simulink library "BPN_lib"  (Simulink 7.4)
settings: Solver=ode45  StartTime=0.0  StopTime=10.0  RelTol=1e-3
values from neighbouring files (symbols this model uses):
  BPNc_fac_ChaPowCurLim = mpt.Parameter    [BPN_CAL.m]
  BPNc_fac_DchPowCurLim = mpt.Parameter    [BPN_CAL.m]
  BPNc_i2_ContiChaCurLim_Max = mpt.Parameter    [BPN_CAL.m]
  BPNc_i2_ContiDchCurLim_Max = mpt.Parameter    [BPN_CAL.m]
  BPNc_i_ContiChaCurLim_Max = mpt.Parameter    [BPN_CAL.m]
  BPNc_i_ContiDchCurLim_Max = mpt.Parameter    [BPN_CAL.m]
  BPNc_i_NorChaCurLim_Max = mpt.Parameter    [BPN_CAL.m]
  BPNc_i_NorDchCurLim_Max = mpt.Parameter    [BPN_CAL.m]
  BPNc_i_PackCurMeasAlwd = mpt.Parameter    [BPN_CAL.m]
  BPNc_i_SafeChaCurLim_Max = mpt.Parameter    [BPN_CAL.m]
  BPNc_i_SafeDchCurLim_Max = mpt.Parameter    [BPN_CAL.m]
  BPNc_pct_CurLimFac_warn = mpt.Parameter    [BPN_CAL.m]
  BPNc_pct_PackSocOver_fatal = mpt.Parameter    [BPN_CAL.m]
  BPNc_pct_PackSocOver_fault = mpt.Parameter    [BPN_CAL.m]
  BPNc_pct_PackSocOver_warn = mpt.Parameter    [BPN_CAL.m]
  BPNc_pct_PackSocUnder_fatal = mpt.Parameter    [BPN_CAL.m]
  BPNc_pct_PackSocUnder_fault = mpt.Parameter    [BPN_CAL.m]
  BPNc_pct_PackSocUnder_warn = mpt.Parameter    [BPN_CAL.m]
  BPNc_pct_PowLimfac_fatal = mpt.Parameter    [BPN_CAL.m]
  BPNc_pct_PowLimfac_warn = mpt.Parameter    [BPN_CAL.m]
  BPNc_r_CtrRes_fault = mpt.Parameter    [BPN_CAL.m]
  BPNc_r_PackInResThrld = mpt.Parameter    [BPN_CAL.m]
  BPNc_t_PackTemp_Mean = mpt.Parameter    [BPN_CAL.m]
  BPNc_v_CellVoltDif_fault = mpt.Parameter    [BPN_CAL.m]
  BPNc_v_CellVoltDif_warn = mpt.Parameter    [BPN_CAL.m]
  BPNc_v_CellVoltOver_fatal = mpt.Parameter    [BPN_CAL.m]
  BPNc_v_CellVoltOver_fault = mpt.Parameter    [BPN_CAL.m]
  BPNc_v_CellVoltOver_warn = mpt.Parameter    [BPN_CAL.m]
  BPNc_v_CellVoltUnder_fatal = mpt.Parameter    [BPN_CAL.m]
  BPNc_v_CellVoltUnder_fault = mpt.Parameter    [BPN_CAL.m]
  BPNc_v_CellVoltUnder_warn = mpt.Parameter    [BPN_CAL.m]
  BPNc_v_LowOPerVolt = mpt.Parameter    [BPN_CAL.m]
  BPNc_v_PackVoltDrop_fatal = mpt.Parameter    [BPN_CAL.m]
  BPNc_v_PackVoltOver_fatal = mpt.Parameter    [BPN_CAL.m]
  BPNc_v_PackVoltOver_fault = mpt.Parameter    [BPN_CAL.m]
  BPNc_v_PackVoltOver_warn = mpt.Parameter    [BPN_CAL.m]
  BPNc_v_PackVoltUnder_fatal = mpt.Parameter    [BPN_CAL.m]
  BPNc_v_PackVoltUnder_fault = mpt.Parameter    [BPN_CAL.m]
  BPNc_v_PackVoltUnder_warn = mpt.Parameter    [BPN_CAL.m]
  BPNc_v_VoltDifThrld = mpt.Parameter    [BPN_CAL.m]
  BPNy_DiagAcvnCtlCtrSt = mpt.Parameter    [BPN_CAL.m]
  BPNz_DiagAcvnCtlId = mpt.Parameter    [BPN_CAL.m]
  BSCx_BCU_State = mpt.Parameter    [BPN_CAL.m]
undefined symbols (not defined in the file or in its folder): BMS_Const_TickTm_s, BPNm_mode_DiaCtlAcv, PACK_Const_CellNumOfMdl, PACK_Const_MdlNumOfPack
libraries: Defined_Functionality x12, simulink x4
(part 2 of 2)

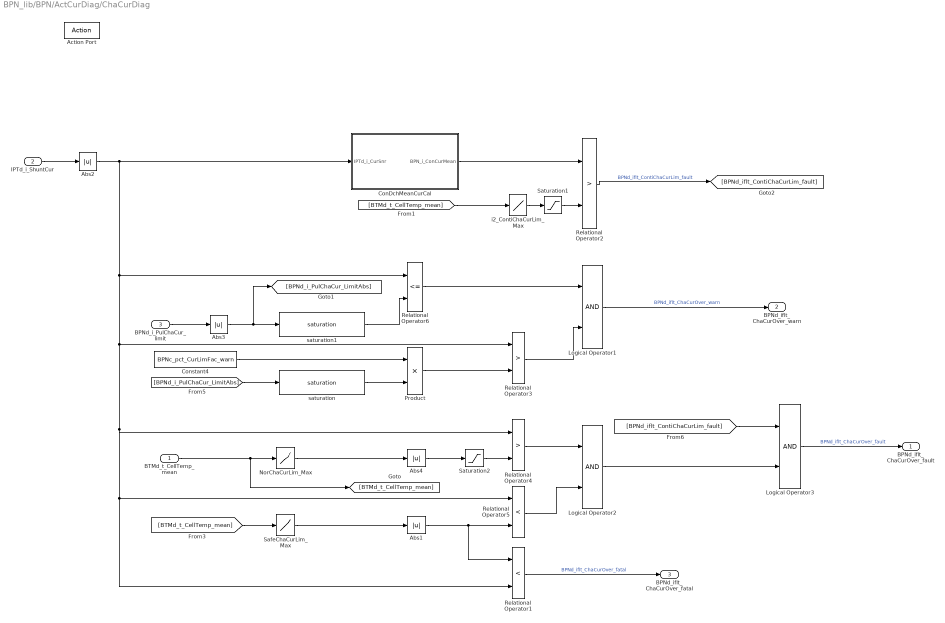
== system BPN_lib/BPN/ActCurDiag/ChaCurDiag ==
  BTMd_t_CellTemp_mean : Inport
  IPTd_i_ShuntCur : Inport  Port=2
  BPNd_i_PulChaCur_limit : Inport  Port=3
  Action Port : ActionPort
  Abs1 : Abs  OutDataType=fixdt(1, 16)  OutScaling=2^0
  Abs2 : Abs
  Abs3 : Abs
  Abs4 : Abs  OutDataType=fixdt(1, 16)  OutScaling=2^0
  ConDchMeanCurCal : Subsystem
  Constant4 : Constant  Value=BPNc_pct_CurLimFac_warn
  Logical Operator1 : Logic  AllPortsSameDT=off  OutDataTypeMode=boolean  OutDataTypeStr=boolean
  Logical Operator2 : Logic  AllPortsSameDT=off  OutDataTypeMode=boolean  OutDataTypeStr=boolean
  Logical Operator3 : Logic  AllPortsSameDT=off  OutDataTypeMode=boolean  OutDataTypeStr=boolean
  NorChaCurLim_Max : Lookup  InputValues=BPNc_t_PackTemp_Mean  Table=BPNc_i_NorChaCurLim_Max  LookUpMeth=Interpolation-Use End Values
  Product : Product  RndMeth=Zero
  Relational Operator1 : RelationalOperator  Operator=<  LogicOutDataTypeMode=boolean  OutDataTypeStr=boolean
  Relational Operator2 : RelationalOperator  Operator=>  LogicOutDataTypeMode=boolean  OutDataTypeStr=boolean
  Relational Operator3 : RelationalOperator  Operator=>  LogicOutDataTypeMode=boolean  OutDataTypeStr=boolean
  Relational Operator4 : RelationalOperator  Operator=>  LogicOutDataTypeMode=boolean  OutDataTypeStr=boolean
  Relational Operator5 : RelationalOperator  Operator=<  LogicOutDataTypeMode=boolean  OutDataTypeStr=boolean
  Relational Operator6 : RelationalOperator  Operator=<=  LogicOutDataTypeMode=boolean  OutDataTypeStr=boolean
  SafeChaCurLim_Max : Lookup  InputValues=BPNc_t_PackTemp_Mean  Table=BPNc_i_SafeChaCurLim_Max  LookUpMeth=Interpolation-Use End Values
  Saturation1 : Saturate  UpperLimit=46000  LowerLimit=100
  Saturation2 : Saturate  UpperLimit=300  LowerLimit=15
  i2_ContiChaCurLim_Max : Lookup  InputValues=BPNc_t_PackTemp_Mean  Table=BPNc_i2_ContiChaCurLim_Max  LookUpMeth=Interpolation-Use End Values
  saturation : Defined_Functionality/saturation  SystemSampleTime=-1  upper_limit=300  lower_limit=15
      settings: AttributesFormatString=[UPPER_LIMIT=%<upper_limit>]\n[LOWER_LIMIT=%<lower_limit>]
  saturation1 : Defined_Functionality/saturation  SystemSampleTime=-1  upper_limit=500  lower_limit=15
      settings: AttributesFormatString=[UPPER_LIMIT=%<upper_limit>]\n[LOWER_LIMIT=%<lower_limit>]
  BPNd_iflt_ChaCurOver_fault : Outport
  BPNd_iflt_ChaCurOver_warn : Outport  Port=2
  BPNd_iflt_ChaCurOver_fatal : Outport  Port=3
  wires:
  Abs2/1 -> Relational Operator6/1, Relational Operator3/1, Relational Operator1/2, Relational Operator5/1, Relational Operator4/1, ConDchMeanCurCal/1(IPTd_i_CurSnr)
  [BPNd_iflt_ContiChaCurLim_fault] -> Logical Operator3/1
  Logical Operator3/1 -> BPNd_iflt_ChaCurOver_fault/1  "BPNd_iflt_ChaCurOver_fault"
  Logical Operator2/1 -> Logical Operator3/2
  Relational Operator2/1 -> [BPNd_iflt_ContiChaCurLim_fault]  "BPNd_iflt_ContiChaCurLim_fault"
  Abs1/1 -> Relational Operator5/2, Relational Operator1/1
  Abs4/1 -> Saturation2/1
  saturation1/1 -> Relational Operator6/2
  Saturation2/1 -> Relational Operator4/2
  Saturation1/1 -> Relational Operator2/2
  saturation/1 -> Product/2
  ConDchMeanCurCal/1(BPN_i_ConCurMean) -> Relational Operator2/1
  Relational Operator5/1 -> Logical Operator2/2
  Relational Operator4/1 -> Logical Operator2/1
  SafeChaCurLim_Max/1 -> Abs1/1
  Logical Operator1/1 -> BPNd_iflt_ChaCurOver_warn/1  "BPNd_iflt_ChaCurOver_warn"
  Relational Operator3/1 -> Logical Operator1/2
  Relational Operator6/1 -> Logical Operator1/1
  [BPNd_i_PulChaCur_LimitAbs] -> saturation/1
  Abs3/1 -> saturation1/1, [BPNd_i_PulChaCur_LimitAbs]
  Product/1 -> Relational Operator3/2
  Constant4/1 -> Product/1
  BPNd_i_PulChaCur_limit/1 -> Abs3/1
  [BTMd_t_CellTemp_mean] -> SafeChaCurLim_Max/1
  [BTMd_t_CellTemp_mean] -> i2_ContiChaCurLim_Max/1
  BTMd_t_CellTemp_mean/1 -> [BTMd_t_CellTemp_mean], NorChaCurLim_Max/1
  NorChaCurLim_Max/1 -> Abs4/1
  IPTd_i_ShuntCur/1 -> Abs2/1
  i2_ContiChaCurLim_Max/1 -> Saturation1/1
  Relational Operator1/1 -> BPNd_iflt_ChaCurOver_fatal/1  "BPNd_iflt_ChaCurOver_fatal"

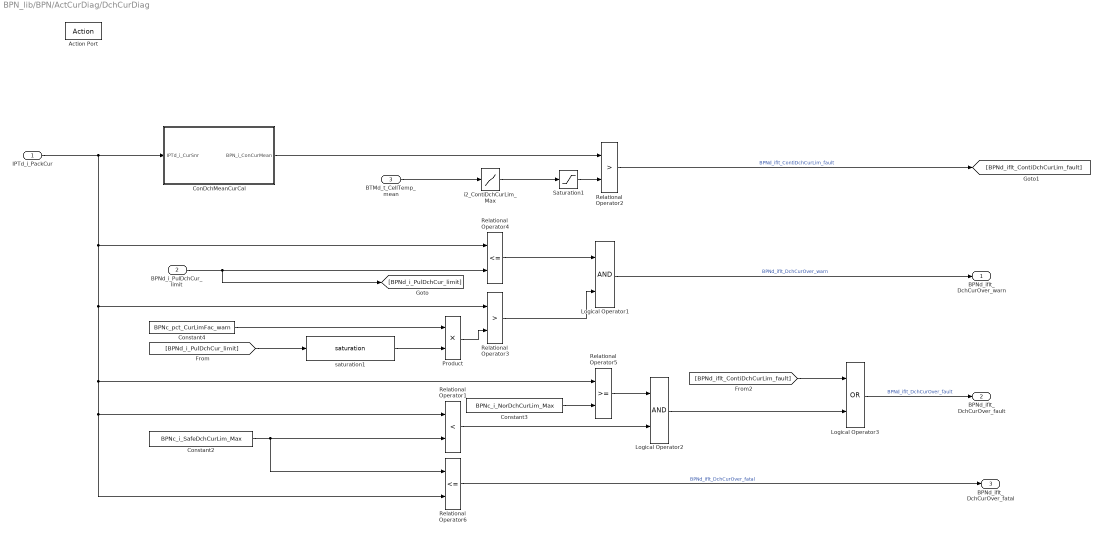
== system BPN_lib/BPN/ActCurDiag/DchCurDiag ==
  IPTd_i_PackCur : Inport  DataType=single  OutDataTypeStr=single
  BPNd_i_PulDchCur_limit : Inport  Port=2
  BTMd_t_CellTemp_mean : Inport  Port=3
  Action Port : ActionPort
  ConDchMeanCurCal : Subsystem
  Constant2 : Constant  Value=BPNc_i_SafeDchCurLim_Max  OutDataTypeMode=single  OutDataTypeStr=single
  Constant3 : Constant  Value=BPNc_i_NorDchCurLim_Max  OutDataTypeMode=single  OutDataTypeStr=single
  Constant4 : Constant  Value=BPNc_pct_CurLimFac_warn
  Logical Operator1 : Logic  AllPortsSameDT=off  OutDataTypeMode=boolean  OutDataTypeStr=boolean
  Logical Operator2 : Logic  AllPortsSameDT=off  OutDataTypeMode=boolean  OutDataTypeStr=boolean
  Logical Operator3 : Logic  Operator=OR  AllPortsSameDT=off  OutDataTypeMode=boolean  OutDataTypeStr=boolean
  Product : Product  RndMeth=Zero
  Relational Operator1 : RelationalOperator  Operator=<  LogicOutDataTypeMode=boolean  OutDataTypeStr=boolean
  Relational Operator2 : RelationalOperator  Operator=>  LogicOutDataTypeMode=boolean  OutDataTypeStr=boolean
  Relational Operator3 : RelationalOperator  Operator=>  LogicOutDataTypeMode=boolean  OutDataTypeStr=boolean
  Relational Operator4 : RelationalOperator  Operator=<=  LogicOutDataTypeMode=boolean  OutDataTypeStr=boolean
  Relational Operator5 : RelationalOperator  LogicOutDataTypeMode=boolean  OutDataTypeStr=boolean
  Relational Operator6 : RelationalOperator  Operator=<=  LogicOutDataTypeMode=boolean  OutDataTypeStr=boolean
  Saturation1 : Saturate  UpperLimit=90000  LowerLimit=5
  i2_ContiDchCurLim_Max : Lookup  InputValues=BPNc_t_PackTemp_Mean  Table=BPNc_i2_ContiDchCurLim_Max  LookUpMeth=Interpolation-Use End Values
  saturation1 : Defined_Functionality/saturation  SystemSampleTime=-1  upper_limit=300  lower_limit=15
      settings: AttributesFormatString=[UPPER_LIMIT=%<upper_limit>]\n[LOWER_LIMIT=%<lower_limit>]
  BPNd_iflt_DchCurOver_warn : Outport
  BPNd_iflt_DchCurOver_fault : Outport  Port=2
  BPNd_iflt_DchCurOver_fatal : Outport  Port=3
  wires:
  saturation1/1 -> Product/2
  [BPNd_i_PulDchCur_limit] -> saturation1/1
  IPTd_i_PackCur/1 -> Relational Operator6/2, Relational Operator1/1, Relational Operator5/1, Relational Operator3/1, Relational Operator4/1, ConDchMeanCurCal/1(IPTd_i_CurSnr)
  [BPNd_iflt_ContiDchCurLim_fault] -> Logical Operator3/1
  Logical Operator3/1 -> BPNd_iflt_DchCurOver_fault/1  "BPNd_iflt_DchCurOver_fault"
  Logical Operator2/1 -> Logical Operator3/2
  Constant3/1 -> Relational Operator5/2
  Relational Operator2/1 -> [BPNd_iflt_ContiDchCurLim_fault]  "BPNd_iflt_ContiDchCurLim_fault"
  ConDchMeanCurCal/1(BPN_i_ConCurMean) -> Relational Operator2/1
  Saturation1/1 -> Relational Operator2/2
  Relational Operator6/1 -> BPNd_iflt_DchCurOver_fatal/1  "BPNd_iflt_DchCurOver_fatal"
  Relational Operator1/1 -> Logical Operator2/2
  Relational Operator5/1 -> Logical Operator2/1
  Constant2/1 -> Relational Operator6/1, Relational Operator1/2
  Logical Operator1/1 -> BPNd_iflt_DchCurOver_warn/1  "BPNd_iflt_DchCurOver_warn"
  Relational Operator3/1 -> Logical Operator1/2
  Relational Operator4/1 -> Logical Operator1/1
  BPNd_i_PulDchCur_limit/1 -> [BPNd_i_PulDchCur_limit], Relational Operator4/2
  Product/1 -> Relational Operator3/2
  Constant4/1 -> Product/1
  i2_ContiDchCurLim_Max/1 -> Saturation1/1
  BTMd_t_CellTemp_mean/1 -> i2_ContiDchCurLim_Max/1

== system BPN_lib/BPN/ActCurDiag/Subsystem ==
  BPNd_i_PulDchCur_limit : Inport
  BPNd_i_PulChaCur_limit : Inport  Port=2
  Abs : Abs  OutDataType=fixdt(1, 16)  OutScaling=2^0
  Bus Creator : BusCreator  Inputs=2
  Bus Creator1 : BusCreator  Inputs=2
  MinMax : MinMax  Function=max
  MinMax1 : MinMax
  Selector : Selector  InputPortWidth=11  IndexOptions=Index vector (dialog)  Indices=2:11  OutputSizes=1
  Selector1 : Selector  InputPortWidth=11  IndexOptions=Index vector (dialog)  Indices=2:11  OutputSizes=1
  Unit Delay : UnitDelay  SampleTime=-1
  Unit Delay1 : UnitDelay  SampleTime=-1
  BPN_i_PulDchCur_limit : Outport
  BPN_i_PulChaCur_LimitAbs : Outport  Port=2
  wires:
  Abs/1 -> BPN_i_PulChaCur_LimitAbs/1
  MinMax1/1 -> Abs/1
  MinMax/1 -> BPN_i_PulDchCur_limit/1
  BPNd_i_PulChaCur_limit/1 -> Bus Creator1/2
  Unit Delay1/1 -> Bus Creator1/1
  Bus Creator1/1 -> Selector1/1
  BPNd_i_PulDchCur_limit/1 -> Bus Creator/2
  Unit Delay/1 -> Bus Creator/1
  Bus Creator/1 -> Selector/1
  Selector1/1 -> MinMax1/1, Unit Delay1/1
  Selector/1 -> MinMax/1, Unit Delay/1

== system BPN_lib/BPN/ActPowDiag/PulChaPower_Diagnosic ==
  BPNd_pow_PackActPower : Inport
  BPNd_pow_PulChaPower_limit : Inport  Port=2
  Action Port : ActionPort
  Abs : Abs
  Abs1 : Abs
  Constant2 : Constant  Value=BPNc_pct_PowLimfac_warn
  Constant3 : Constant  Value=BPNc_pct_PowLimfac_fatal
  Logical Operator1 : Logic  AllPortsSameDT=off  OutDataTypeMode=boolean  OutDataTypeStr=boolean
  Product2 : Product  RndMeth=Zero
  Product3 : Product  RndMeth=Zero
  Relational Operator2 : RelationalOperator  Operator=<  LogicOutDataTypeMode=boolean  OutDataTypeStr=boolean
  Relational Operator3 : RelationalOperator  LogicOutDataTypeMode=boolean  OutDataTypeStr=boolean
  Relational Operator4 : RelationalOperator  Operator=<=  LogicOutDataTypeMode=boolean  OutDataTypeStr=boolean
  Relational Operator6 : RelationalOperator  Operator=>  LogicOutDataTypeMode=boolean  OutDataTypeStr=boolean
  saturation : Defined_Functionality/saturation  SystemSampleTime=-1  upper_limit=500000  lower_limit=10000
      settings: AttributesFormatString=[UPPER_LIMIT=%<upper_limit>]\n[LOWER_LIMIT=%<lower_limit>]
  signal_debug : Defined_Functionality/signal_debug  SystemSampleTime=-1  debug_switch=BPNc_dbgsw_PulChaPowOverWarn  debug_value=IPTc_dbgval__PulChaPowOverWarn
      settings: AttributesFormatString=[SWITCH=%<debug_switch>]\n[VALUE=%<debug_value>]
  signal_debug1 : Defined_Functionality/signal_debug  SystemSampleTime=-1  debug_switch=BPNc_dbgsw_PulChaPowOverFault  debug_value=IPTc_dbgval__PulChaPowOverFault
      settings: AttributesFormatString=[SWITCH=%<debug_switch>]\n[VALUE=%<debug_value>]
  signal_debug2 : Defined_Functionality/signal_debug  SystemSampleTime=-1  debug_switch=BPNc_dbgsw_PulChaPowOverFatal  debug_value=IPTc_dbgval__PulChaPowOverFatal
      settings: AttributesFormatString=[SWITCH=%<debug_switch>]\n[VALUE=%<debug_value>]
  BPNd_iflt_PulChaPowOver_warn : Outport
  BPNd_iflt_PulChaPowOver_fault : Outport  Port=2
  BPNd_iflt_PulChaPowOver_fatal : Outport  Port=3
  wires:
  Product3/1 -> Relational Operator4/1, Relational Operator2/2
  saturation/1 -> [BPNd_pow_PulChaPower_LimitAbs], Product2/2
  signal_debug2/1 -> BPNd_iflt_PulChaPowOver_fatal/1  "BPNd_iflt_PulChaPowOver_fatal"
  signal_debug1/1 -> BPNd_iflt_PulChaPowOver_fault/1  "BPNd_iflt_PulChaPowOver_fault"
  signal_debug/1 -> BPNd_iflt_PulChaPowOver_warn/1  "BPNd_iflt_PulChaPowOver_warn"
  Product2/1 -> Relational Operator3/2
  Abs1/1 -> saturation/1
  Constant2/1 -> Product2/1
  Logical Operator1/1 -> signal_debug1/1
  Relational Operator2/1 -> Logical Operator1/2
  Relational Operator6/1 -> Logical Operator1/1
  [BPNd_pow_PulChaPower_LimitAbs] -> Relational Operator6/2
  Relational Operator3/1 -> signal_debug/1
  Relational Operator4/1 -> signal_debug2/1
  Abs/1 -> Relational Operator3/1, Relational Operator6/1, Relational Operator4/2, Relational Operator2/1
  Constant3/1 -> Product3/2
  [BPNd_pow_PulChaPower_LimitAbs] -> Product3/1
  BPNd_pow_PulChaPower_limit/1 -> Abs1/1
  BPNd_pow_PackActPower/1 -> Abs/1

== system BPN_lib/BPN/ActPowDiag/PulDchPower_Diagnosic ==
  BPNd_pow_PulDchPower_limit : Inport
  BPNd_pow_PackActPower : Inport  Port=2
  Action Port : ActionPort
  Constant1 : Constant  Value=BPNc_pct_PowLimfac_warn  VectorParams1D=off
  Constant2 : Constant  Value=BPNc_pct_PowLimfac_fatal
  Logical Operator : Logic  AllPortsSameDT=off  OutDataTypeMode=boolean  OutDataTypeStr=boolean
  Product1 : Product  RndMeth=Zero
  Product2 : Product  RndMeth=Zero
  Relational Operator1 : RelationalOperator  Operator=<  LogicOutDataTypeMode=boolean  OutDataTypeStr=boolean
  Relational Operator2 : RelationalOperator  Operator=<  LogicOutDataTypeMode=boolean  OutDataTypeStr=boolean
  Relational Operator4 : RelationalOperator  Operator=>  LogicOutDataTypeMode=boolean  OutDataTypeStr=boolean
  Relational Operator6 : RelationalOperator  Operator=<  LogicOutDataTypeMode=boolean  OutDataTypeStr=boolean
  accumulation1 : Defined_Functionality/accumulation  SystemSampleTime=-1  Num_Threshold_Up=200  Num_Threshold_Down=0  Inc=1  Dec=0
      settings: AttributesFormatString=[THRESHOLD_UP=%<Num_Threshold_Up>]\n[THRESHOLD_DOWN=%<Num_Threshold_Down>]\n[INCREMENT=%<Inc>]\n[DECREMENT=%<Dec>]
  saturation : Defined_Functionality/saturation  SystemSampleTime=-1  upper_limit=500000  lower_limit=10000
      settings: AttributesFormatString=[UPPER_LIMIT=%<upper_limit>]\n[LOWER_LIMIT=%<lower_limit>]
  BPNd_iflt_PulDchPowOver_warn : Outport
  BPNd_iflt_PulDchPowOver_fault : Outport  Port=2
  BPNd_iflt_PulDchPowOver_fatal : Outport  Port=3
  wires:
  Product2/1 -> Relational Operator6/1, Relational Operator1/2
  saturation/1 -> [BPNd_pow_PulDchPower_LimitSat], Product1/1
  Constant1/1 -> Product1/2
  BPNd_pow_PulDchPower_limit/1 -> saturation/1
  accumulation1/1 -> BPNd_iflt_PulDchPowOver_fault/1  "BPNd_iflt_PulDchPowOver_fault"
  Relational Operator4/1 -> Logical Operator/1
  Relational Operator2/1 -> BPNd_iflt_PulDchPowOver_warn/1  "BPNd_iflt_PulDchPowOver_warn"
  Relational Operator6/1 -> BPNd_iflt_PulDchPowOver_fatal/1  "BPNd_iflt_PulDchPowOver_fatal"
  Logical Operator/1 -> accumulation1/1
  Relational Operator1/1 -> Logical Operator/2
  Constant2/1 -> Product2/2
  [BPNd_pow_PulDchPower_LimitSat] -> Product2/1
  [BPNd_pow_PulDchPower_LimitSat] -> Relational Operator4/2
  BPNd_pow_PackActPower/1 -> Relational Operator2/2, Relational Operator4/1, Relational Operator6/2, Relational Operator1/1
  Product1/1 -> Relational Operator2/1

== system BPN_lib/BPN/CellVoltDiag/delay ==
  In1 : Inport
  In2 : Inport  Port=2
  Unit Delay1 : UnitDelay  SampleTime=-1
  Unit Delay2 : UnitDelay  SampleTime=-1
  Out1 : Outport
  Out2 : Outport  Port=2
  wires:
  Unit Delay2/1 -> Out2/1
  Unit Delay1/1 -> Out1/1
  In2/1 -> Unit Delay2/1
  In1/1 -> Unit Delay1/1

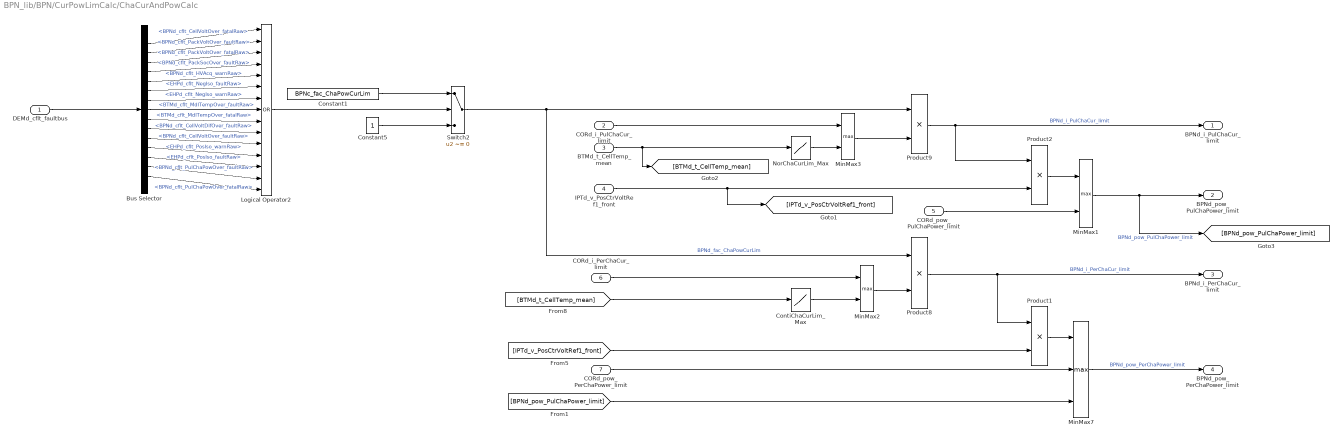
== system BPN_lib/BPN/CurPowLimCalc/ChaCurAndPowCalc ==
  DEMd_cflt_faultbus : Inport  OutDataType=fixdt(1, 16)  OutScaling=2^0
  CORd_i_PulChaCur_limit : Inport  Port=2
  BTMd_t_CellTemp_mean : Inport  Port=3
  IPTd_v_PosCtrVoltRef1_front : Inport  Port=4
  CORd_pow_PulChaPower_limit : Inport  Port=5
  CORd_i_PerChaCur_limit : Inport  Port=6
  CORd_pow_PerChaPower_limit : Inport  Port=7
  Bus Selector : BusSelector  OutputSignals=BPN_Fault_Bus.BPNd_cflt_CellVoltOver_fatalRaw,BPN_Fault_Bus.BPNd_cflt_PackVoltOver_faultRaw,BPN_Fault_Bus.BPNd_cflt_PackVoltOver_fatalRaw,BPN_Fault_Bus.BPNd_cflt_PackSocOver_faultRaw,BPN_Fault_Bus.BPNd_cflt_HVAcq_warnRaw,EHP_Fault_Bus.EHPd_cflt_NegIso_faultRaw,EHP_Fault_Bus.EHPd_cflt_NegIso_warnRaw,BTM_Fault_Bus.BTMd_cflt_MdlTempOver_faultRaw,BTM_Fault_Bus.BTMd_cflt_MdlTempOver_fatalRaw,BPN_Fault_Bus.BPNd_cflt_CellVoltDifOver_faultRaw,BPN_Fault_Bus.BPNd_cflt_CellVoltOver_faultRaw,EHP_Fault_Bus.EHPd_cflt_PosIso_warnRaw,EHP_Fault_Bus.EHPd_cflt_PosIso_faultRaw,BPN_Fault_Bus.BPNd_cflt_PulChaPowOver_faultRaw,BPN_Fault_Bus.BPNd_cflt_PulChaPowOver_fatalRaw
  Constant1 : Constant  Value=BPNc_fac_ChaPowCurLim  OutDataTypeMode=single  OutDataTypeStr=single
  Constant5 : Constant  OutDataTypeMode=single  OutDataType=fixdt(1, 16)  OutScaling=2^0  OutDataTypeStr=single
  ContiChaCurLim_Max : Lookup  InputValues=BPNc_t_PackTemp_Mean  Table=BPNc_i_ContiChaCurLim_Max  LookUpMeth=Interpolation-Use End Values
  Logical Operator2 : Logic  Operator=OR  Inputs=15  AllPortsSameDT=off  OutDataTypeMode=boolean  LogicDataType=fixdt(0, 8)  OutDataTypeStr=boolean
  MinMax1 : MinMax  Function=max  Inputs=2  OutDataTypeMode=single  OutDataTypeStr=single
  MinMax2 : MinMax  Function=max  Inputs=2  OutDataTypeMode=single  OutDataTypeStr=single
  MinMax3 : MinMax  Function=max  Inputs=2  OutDataTypeMode=single  OutDataTypeStr=single
  MinMax7 : MinMax  Function=max  Inputs=3  OutDataTypeMode=single  OutDataTypeStr=single
  NorChaCurLim_Max : Lookup  InputValues=BPNc_t_PackTemp_Mean  Table=BPNc_i_NorChaCurLim_Max  LookUpMeth=Interpolation-Use End Values
  Product{1..2,8..9} (4 alike) : Product  RndMeth=Zero
  Switch2 : Switch  Criteria=u2 ~= 0  Threshold=1  OutDataType=fixdt(1, 16)  OutScaling=2^0
  BPNd_i_PulChaCur_limit : Outport
  BPNd_pow_PulChaPower_limit : Outport  Port=2
  BPNd_i_PerChaCur_limit : Outport  Port=3
  BPNd_pow_PerChaPower_limit : Outport  Port=4
  wires:
  DEMd_cflt_faultbus/1 -> Bus Selector/1
  Bus Selector/15 -> Logical Operator2/15  "<BPNd_cflt_PulChaPowOver_fatalRaw>"
  Bus Selector/14 -> Logical Operator2/14  "<BPNd_cflt_PulChaPowOver_faultRaw>"
  Bus Selector/13 -> Logical Operator2/13  "<EHPd_cflt_PosIso_faultRaw>"
  Bus Selector/12 -> Logical Operator2/12  "<EHPd_cflt_PosIso_warnRaw>"
  Bus Selector/11 -> Logical Operator2/11  "<BPNd_cflt_CellVoltOver_faultRaw>"
  Bus Selector/10 -> Logical Operator2/10  "<BPNd_cflt_CellVoltDifOver_faultRaw>"
  Bus Selector/9 -> Logical Operator2/9  "<BTMd_cflt_MdlTempOver_fatalRaw>"
  Bus Selector/8 -> Logical Operator2/8  "<BTMd_cflt_MdlTempOver_faultRaw>"
  Bus Selector/7 -> Logical Operator2/7  "<EHPd_cflt_NegIso_warnRaw>"
  Bus Selector/6 -> Logical Operator2/6  "<EHPd_cflt_NegIso_faultRaw>"
  Bus Selector/5 -> Logical Operator2/5  "<BPNd_cflt_HVAcq_warnRaw>"
  Bus Selector/4 -> Logical Operator2/4  "<BPNd_cflt_PackSocOver_faultRaw>"
  Bus Selector/3 -> Logical Operator2/3  "<BPNd_cflt_PackVoltOver_fatalRaw>"
  Bus Selector/2 -> Logical Operator2/2  "<BPNd_cflt_PackVoltOver_faultRaw>"
  Bus Selector/1 -> Logical Operator2/1  "<BPNd_cflt_CellVoltOver_fatalRaw>"
  [BPNd_pow_PulChaPower_limit] -> MinMax7/3
  MinMax7/1 -> BPNd_pow_PerChaPower_limit/1  "BPNd_pow_PerChaPower_limit"
  CORd_pow_PerChaPower_limit/1 -> MinMax7/2
  Product1/1 -> MinMax7/1
  [IPTd_v_PosCtrVoltRef1_front] -> Product1/2
  MinMax2/1 -> Product8/2
  CORd_i_PerChaCur_limit/1 -> MinMax2/1
  MinMax1/1 -> [BPNd_pow_PulChaPower_limit], BPNd_pow_PulChaPower_limit/1  "BPNd_pow_PulChaPower_limit"
  Product2/1 -> MinMax1/1
  CORd_pow_PulChaPower_limit/1 -> MinMax1/2
  NorChaCurLim_Max/1 -> MinMax3/2
  CORd_i_PulChaCur_limit/1 -> MinMax3/1
  Constant1/1 -> Switch2/1
  Constant5/1 -> Switch2/3
  Logical Operator2/1 -> Switch2/2
  ContiChaCurLim_Max/1 -> MinMax2/2
  IPTd_v_PosCtrVoltRef1_front/1 -> [IPTd_v_PosCtrVoltRef1_front], Product2/2
  Product8/1 -> Product1/1, BPNd_i_PerChaCur_limit/1  "BPNd_i_PerChaCur_limit"
  Product9/1 -> Product2/1, BPNd_i_PulChaCur_limit/1  "BPNd_i_PulChaCur_limit"
  MinMax3/1 -> Product9/2
  BTMd_t_CellTemp_mean/1 -> [BTMd_t_CellTemp_mean], NorChaCurLim_Max/1
  Switch2/1 -> Product8/1, Product9/1  "BPNd_fac_ChaPowCurLim"
  [BTMd_t_CellTemp_mean] -> ContiChaCurLim_Max/1

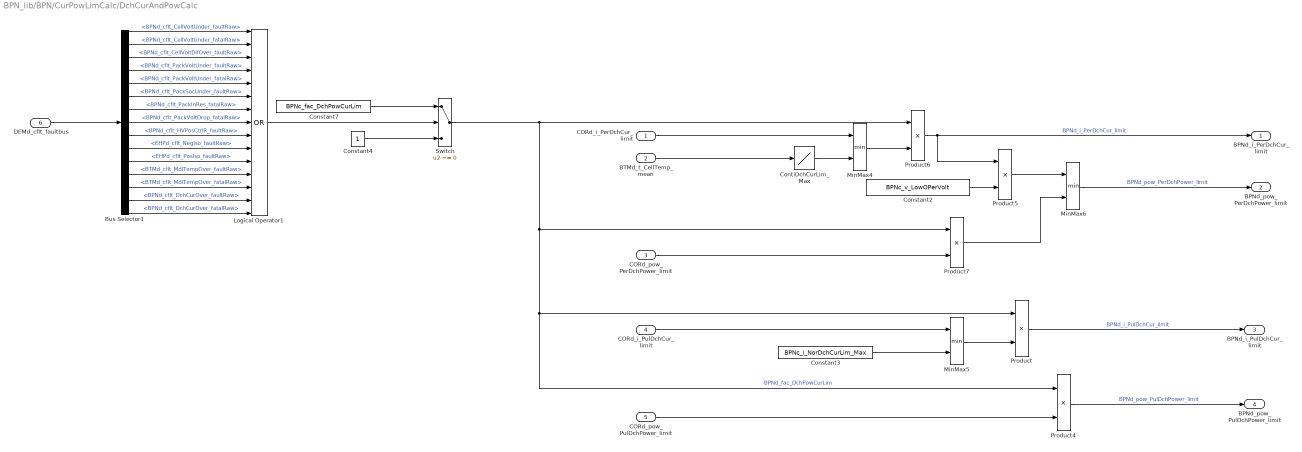
== system BPN_lib/BPN/CurPowLimCalc/DchCurAndPowCalc ==
  CORd_i_PerDchCur_limit : Inport
  BTMd_t_CellTemp_mean : Inport  Port=2
  CORd_pow_PerDchPower_limit : Inport  Port=3
  CORd_i_PulDchCur_limit : Inport  Port=4  DataType=single  OutDataTypeStr=single
  CORd_pow_PulDchPower_limit : Inport  Port=5
  DEMd_cflt_faultbus : Inport  Port=6  OutDataType=fixdt(1, 16)  OutScaling=2^0
  Bus Selector1 : BusSelector  OutputSignals=BPN_Fault_Bus.BPNd_cflt_CellVoltUnder_faultRaw,BPN_Fault_Bus.BPNd_cflt_CellVoltUnder_fatalRaw,BPN_Fault_Bus.BPNd_cflt_CellVoltDifOver_faultRaw,BPN_Fault_Bus.BPNd_cflt_PackVoltUnder_faultRaw,BPN_Fault_Bus.BPNd_cflt_PackVoltUnder_fatalRaw,BPN_Fault_Bus.BPNd_cflt_PackSocUnder_faultRaw,BPN_Fault_Bus.BPNd_cflt_PackInRes_fatalRaw,BPN_Fault_Bus.BPNd_cflt_PackVoltDrop_fatalRaw,BPN_Fault_Bus.BPNd_cflt_HVPosCtrlR_faultRaw,EHP_Fault_Bus.EHPd_cflt_NegIso_faultRaw,EHP_Fault_Bus.EHPd_cflt_PosIso_faultRaw,BTM_Fault_Bus.BTMd_cflt_MdlTempOver_faultRaw,BTM_Fault_Bus.BTMd_cflt_MdlTempOver_fatalRaw,BPN_Fault_Bus.BPNd_cflt_DchCurOver_faultRaw,BPN_Fault_Bus.BPNd_cflt_DchCurOver_fatalRaw
  Constant2 : Constant  Value=BPNc_v_LowOPerVolt  OutDataTypeMode=single  OutDataTypeStr=single
  Constant3 : Constant  Value=BPNc_i_NorDchCurLim_Max  OutDataTypeMode=single  OutDataTypeStr=single
  Constant4 : Constant  OutDataTypeMode=single  OutDataType=fixdt(1, 16)  OutScaling=2^0  OutDataTypeStr=single
  Constant7 : Constant  Value=BPNc_fac_DchPowCurLim  OutDataTypeMode=single  OutDataTypeStr=single
  ContiDchCurLim_Max : Lookup  InputValues=BPNc_t_PackTemp_Mean  Table=BPNc_i_ContiDchCurLim_Max  LookUpMeth=Interpolation-Use End Values
  Logical Operator1 : Logic  Operator=OR  Inputs=15  AllPortsSameDT=off  OutDataTypeMode=boolean  LogicDataType=fixdt(0, 8)  OutDataTypeStr=boolean
  MinMax4 : MinMax  Inputs=2  OutDataTypeMode=single  OutDataTypeStr=single
  MinMax5 : MinMax  Inputs=2  OutDataTypeMode=single  OutDataTypeStr=single
  MinMax6 : MinMax  Inputs=2  OutDataTypeMode=single  OutDataTypeStr=single
  Product{,4..7} (5 alike) : Product  RndMeth=Zero
  Switch : Switch  Criteria=u2 ~= 0  Threshold=1  OutDataType=fixdt(1, 16)  OutScaling=2^0
  BPNd_i_PerDchCur_limit : Outport  DataType=single  OutDataTypeStr=single
  BPNd_pow_PerDchPower_limit : Outport  Port=2  DataType=single  OutDataTypeStr=single
  BPNd_i_PulDchCur_limit : Outport  Port=3
  BPNd_pow_PulDchPower_limit : Outport  Port=4
  wires:
  Bus Selector1/15 -> Logical Operator1/15  "<BPNd_cflt_DchCurOver_fatalRaw>"
  Bus Selector1/14 -> Logical Operator1/14  "<BPNd_cflt_DchCurOver_faultRaw>"
  Bus Selector1/13 -> Logical Operator1/13  "<BTMd_cflt_MdlTempOver_fatalRaw>"
  Bus Selector1/12 -> Logical Operator1/12  "<BTMd_cflt_MdlTempOver_faultRaw>"
  Bus Selector1/11 -> Logical Operator1/11  "<EHPd_cflt_PosIso_faultRaw>"
  Bus Selector1/10 -> Logical Operator1/10  "<EHPd_cflt_NegIso_faultRaw>"
  Bus Selector1/9 -> Logical Operator1/9  "<BPNd_cflt_HVPosCtrlR_faultRaw>"
  Bus Selector1/8 -> Logical Operator1/8  "<BPNd_cflt_PackVoltDrop_fatalRaw>"
  Bus Selector1/7 -> Logical Operator1/7  "<BPNd_cflt_PackInRes_fatalRaw>"
  Bus Selector1/6 -> Logical Operator1/6  "<BPNd_cflt_PackSocUnder_faultRaw>"
  Bus Selector1/5 -> Logical Operator1/5  "<BPNd_cflt_PackVoltUnder_fatalRaw>"
  Bus Selector1/4 -> Logical Operator1/4  "<BPNd_cflt_PackVoltUnder_faultRaw>"
  Bus Selector1/3 -> Logical Operator1/3  "<BPNd_cflt_CellVoltDifOver_faultRaw>"
  Bus Selector1/2 -> Logical Operator1/2  "<BPNd_cflt_CellVoltUnder_fatalRaw>"
  Bus Selector1/1 -> Logical Operator1/1  "<BPNd_cflt_CellVoltUnder_faultRaw>"
  CORd_pow_PulDchPower_limit/1 -> Product4/2
  MinMax6/1 -> BPNd_pow_PerDchPower_limit/1  "BPNd_pow_PerDchPower_limit"
  Product5/1 -> MinMax6/1
  Constant2/1 -> Product5/2
  Switch/1 -> Product4/1, Product/1, Product7/1, Product6/1  "BPNd_fac_DchPowCurLim"
  MinMax4/1 -> Product6/2
  Constant4/1 -> Switch/3
  Constant7/1 -> Switch/1
  Logical Operator1/1 -> Switch/2
  Product6/1 -> Product5/1, BPNd_i_PerDchCur_limit/1  "BPNd_i_PerDchCur_limit"
  ContiDchCurLim_Max/1 -> MinMax4/2
  MinMax5/1 -> Product/2
  Constant3/1 -> MinMax5/2
  CORd_i_PerDchCur_limit/1 -> MinMax4/1
  Product7/1 -> MinMax6/2
  CORd_pow_PerDchPower_limit/1 -> Product7/2
  Product/1 -> BPNd_i_PulDchCur_limit/1  "BPNd_i_PulDchCur_limit"
  CORd_i_PulDchCur_limit/1 -> MinMax5/1
  DEMd_cflt_faultbus/1 -> Bus Selector1/1
  BTMd_t_CellTemp_mean/1 -> ContiDchCurLim_Max/1
  Product4/1 -> BPNd_pow_PulDchPower_limit/1  "BPNd_pow_PulDchPower_limit"

== system BPN_lib/BPN/HVCtrResDiag/HVCtrResDiag ==
  IPTd_v_PosCtrVoltRef1_front : Inport
  IPTd_v_PosCtrVoltRef1_back : Inport  Port=2
  IPTd_i_DCLinkCur : Inport  Port=3
  IPTd_v_PosCtrVoltRef2_front : Inport  Port=4
  Enable : EnablePort
  Abs : Abs
  Abs1 : Abs
  Constant : Constant  Value=BPNc_r_CtrRes_fault
  Constant2 : Constant  Value=BPNc_r_CtrRes_fault
  Divide : Product  Inputs=*/
  Divide1 : Product  Inputs=/*
  Relational Operator : RelationalOperator  LogicOutDataTypeMode=boolean  OutDataTypeStr=boolean
  Relational Operator1 : RelationalOperator  LogicOutDataTypeMode=boolean  OutDataTypeStr=boolean
  Subtract : Sum  Inputs=+-
  Subtract1 : Sum  Inputs=+-
  saturation : Defined_Functionality/saturation  SystemSampleTime=-1  upper_limit=360  lower_limit=40
      settings: AttributesFormatString=[UPPER_LIMIT=%<upper_limit>]\n[LOWER_LIMIT=%<lower_limit>]
  BPNd_iflt_HVPosCtrlR_fault : Outport
  BPNd_iflt_HVNegCtrlR_fault : Outport  Port=2  InitialOutput=0
  wires:
  saturation/1 -> Divide1/1, Divide/2
  [IPTd_v_PosCtrVoltRef1_front] -> Subtract1/1
  Abs1/1 -> Divide1/2
  Constant/1 -> Relational Operator/2
  Constant2/1 -> Relational Operator1/2
  Divide1/1 -> Relational Operator1/1
  Subtract1/1 -> Abs1/1
  IPTd_v_PosCtrVoltRef2_front/1 -> Subtract1/2
  IPTd_i_DCLinkCur/1 -> saturation/1
  Relational Operator1/1 -> BPNd_iflt_HVNegCtrlR_fault/1  "BPNd_iflt_HVNegCtrlR_fault"
  Abs/1 -> Divide/1
  Subtract/1 -> Abs/1
  Divide/1 -> Relational Operator/1
  Relational Operator/1 -> BPNd_iflt_HVPosCtrlR_fault/1  "BPNd_iflt_HVPosCtrlR_fault"
  IPTd_v_PosCtrVoltRef1_back/1 -> Subtract/2
  IPTd_v_PosCtrVoltRef1_front/1 -> [IPTd_v_PosCtrVoltRef1_front], Subtract/1

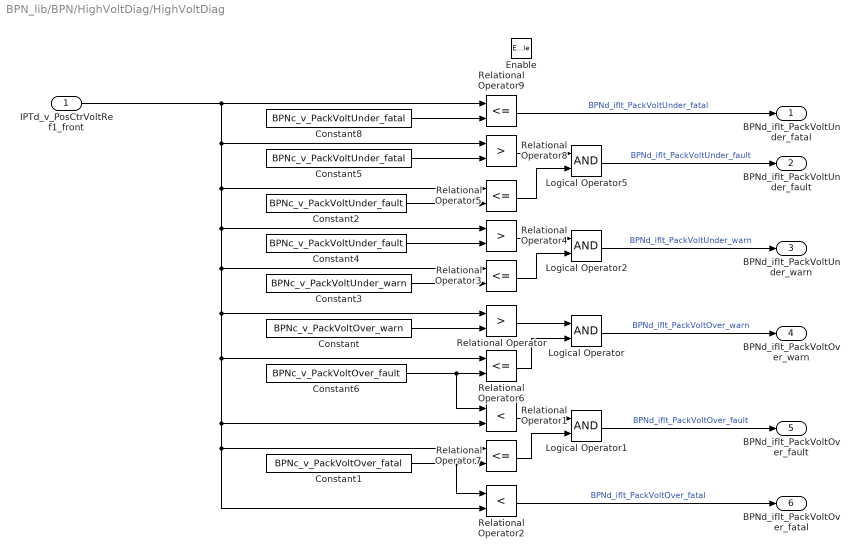
== system BPN_lib/BPN/HighVoltDiag/HighVoltDiag ==
  IPTd_v_PosCtrVoltRef1_front : Inport
  Enable : EnablePort
  Constant : Constant  Value=BPNc_v_PackVoltOver_warn  OutDataTypeMode=single  OutDataTypeStr=single
  Constant1 : Constant  Value=BPNc_v_PackVoltOver_fatal  OutDataTypeMode=single  OutDataTypeStr=single
  Constant2 : Constant  Value=BPNc_v_PackVoltUnder_fault  OutDataTypeMode=single  OutDataTypeStr=single
  Constant3 : Constant  Value=BPNc_v_PackVoltUnder_warn  OutDataTypeMode=single  OutDataTypeStr=single
  Constant4 : Constant  Value=BPNc_v_PackVoltUnder_fault  OutDataTypeMode=single  OutDataTypeStr=single
  Constant5 : Constant  Value=BPNc_v_PackVoltUnder_fatal  OutDataTypeMode=single  OutDataTypeStr=single
  Constant6 : Constant  Value=BPNc_v_PackVoltOver_fault  OutDataTypeMode=single  OutDataTypeStr=single
  Constant8 : Constant  Value=BPNc_v_PackVoltUnder_fatal  OutDataTypeMode=single  OutDataTypeStr=single
  Logical Operator{,1..2,5} (4 alike) : Logic  AllPortsSameDT=off  OutDataTypeMode=boolean  OutDataTypeStr=boolean
  Relational Operator : RelationalOperator  Operator=>  LogicOutDataTypeMode=boolean  OutDataTypeStr=boolean
  Relational Operator1 : RelationalOperator  Operator=<  LogicOutDataTypeMode=boolean  OutDataTypeStr=boolean
  Relational Operator2 : RelationalOperator  Operator=<  LogicOutDataTypeMode=boolean  OutDataTypeStr=boolean
  Relational Operator{3,5..7,9} (5 alike) : RelationalOperator  Operator=<=  LogicOutDataTypeMode=boolean  OutDataTypeStr=boolean
  Relational Operator4 : RelationalOperator  Operator=>  LogicOutDataTypeMode=boolean  OutDataTypeStr=boolean
  Relational Operator8 : RelationalOperator  Operator=>  LogicOutDataTypeMode=boolean  OutDataTypeStr=boolean
  BPNd_iflt_PackVoltUnder_fatal : Outport
  BPNd_iflt_PackVoltUnder_fault : Outport  Port=2
  BPNd_iflt_PackVoltUnder_warn : Outport  Port=3
  BPNd_iflt_PackVoltOver_warn : Outport  Port=4
  BPNd_iflt_PackVoltOver_fault : Outport  Port=5
  BPNd_iflt_PackVoltOver_fatal : Outport  Port=6
  wires:
  IPTd_v_PosCtrVoltRef1_front/1 -> Relational Operator2/2, Relational Operator7/1, Relational Operator1/2, Relational Operator6/1, Relational Operator/1, Relational Operator3/1, Relational Operator4/1, Relational Operator5/1, Relational Operator8/1, Relational Operator9/1
  Constant8/1 -> Relational Operator9/2
  Constant5/1 -> Relational Operator8/2
  Constant2/1 -> Relational Operator5/2
  Constant4/1 -> Relational Operator4/2
  Constant3/1 -> Relational Operator3/2
  Constant/1 -> Relational Operator/2
  Constant6/1 -> Relational Operator1/1, Relational Operator6/2
  Relational Operator/1 -> Logical Operator/1
  Relational Operator6/1 -> Logical Operator/2
  Relational Operator1/1 -> Logical Operator1/1
  Relational Operator7/1 -> Logical Operator1/2
  Constant1/1 -> Relational Operator2/1, Relational Operator7/2
  Relational Operator3/1 -> Logical Operator2/2
  Relational Operator4/1 -> Logical Operator2/1
  Relational Operator8/1 -> Logical Operator5/1
  Relational Operator5/1 -> Logical Operator5/2
  Relational Operator9/1 -> BPNd_iflt_PackVoltUnder_fatal/1  "BPNd_iflt_PackVoltUnder_fatal"
  Logical Operator5/1 -> BPNd_iflt_PackVoltUnder_fault/1  "BPNd_iflt_PackVoltUnder_fault"
  Logical Operator2/1 -> BPNd_iflt_PackVoltUnder_warn/1  "BPNd_iflt_PackVoltUnder_warn"
  Logical Operator1/1 -> BPNd_iflt_PackVoltOver_fault/1  "BPNd_iflt_PackVoltOver_fault"
  Logical Operator/1 -> BPNd_iflt_PackVoltOver_warn/1  "BPNd_iflt_PackVoltOver_warn"
  Relational Operator2/1 -> BPNd_iflt_PackVoltOver_fatal/1  "BPNd_iflt_PackVoltOver_fatal"

== system BPN_lib/BPN/PackInResDiag/PackInResDiag ==
  IPTd_v_CellVolt : Inport
  IPTd_v_PosCtrVoltRef1_front : Inport  Port=2
  BPNd_i_DClinkCurAbs : Inport  Port=3
  Enable : EnablePort
  Constant : Constant  Value=BPNc_r_PackInResThrld
  Divide : Product  Inputs=*/
  Relational Operator : RelationalOperator  LogicOutDataTypeMode=boolean  OutDataTypeStr=boolean
  Subtract : Sum  Inputs=+-
  Sum of Elements : Sum  Inputs=+
  saturation : Defined_Functionality/saturation  SystemSampleTime=-1  upper_limit=300  lower_limit=1
      settings: AttributesFormatString=[UPPER_LIMIT=%<upper_limit>]\n[LOWER_LIMIT=%<lower_limit>]
  BPNd_iflt_PackInRes_fatal : Outport
  wires:
  saturation/1 -> Divide/2
  BPNd_i_DClinkCurAbs/1 -> saturation/1
  Sum of Elements/1 -> Subtract/1
  Subtract/1 -> Divide/1
  Divide/1 -> Relational Operator/1
  Constant/1 -> Relational Operator/2
  Relational Operator/1 -> BPNd_iflt_PackInRes_fatal/1  "BPNd_iflt_PackInRes_fatal"
  IPTd_v_PosCtrVoltRef1_front/1 -> Subtract/2
  IPTd_v_CellVolt/1 -> Sum of Elements/1

== system BPN_lib/BPN/PackVoltDropDiag/PackVoltDropDiag ==
  IPTd_v_PosCtrVoltRef1_front : Inport
  Enable : EnablePort
  Constant1 : Constant  Value=BPNc_v_PackVoltDrop_fatal
  Data Store Memory : DataStoreMemory  DataStoreName=IPTc_v_PosCtrVoltRef1Max_front  ReadBeforeWriteMsg=warning  WriteAfterWriteMsg=warning  WriteAfterReadMsg=warning
  IPTc_v_PosCtrVoltRef1Max_back1 : DataStoreRead  DataStoreName=IPTc_v_PosCtrVoltRef1Max_front  SampleTime=-1
  Logical Operator : Logic  Operator=NOT  AllPortsSameDT=off  OutDataTypeMode=boolean  OutDataTypeStr=boolean
  MaxVoltMemoryMemory : Subsystem
  MinMax : MinMax  Function=max  Inputs=2
  Relational Operator1 : RelationalOperator  LogicOutDataTypeMode=boolean  OutDataTypeStr=boolean
  Subtract1 : Sum  Inputs=+-
  Subtract2 : Sum  Inputs=+-
  Switch : Switch  Criteria=u2 ~= 0
  Unit Delay1 : UnitDelay  SampleTime=-1
  Unit Delay2 : UnitDelay  SampleTime=-1
  BPNd_ilft_PackVoltDrop_fatal : Outport
  wires:
  MinMax/1 -> Subtract1/1, MaxVoltMemoryMemory/1(IPTd_v_PosCtrVoltRef1Max_front)
  [BPNd_ilft_PackVoltDrop_fatal] -> MaxVoltMemoryMemory/Enable
  [BPNd_ilft_PackVoltDrop_fatal] -> Unit Delay2/1
  Logical Operator/1 -> Switch/2
  Unit Delay2/1 -> Logical Operator/1
  Constant1/1 -> Relational Operator1/2
  Relational Operator1/1 -> [BPNd_ilft_PackVoltDrop_fatal], BPNd_ilft_PackVoltDrop_fatal/1  "BPNd_ilft_PackVoltDrop_fatal"
  IPTd_v_PosCtrVoltRef1_front/1 -> Subtract1/2, Subtract2/2, Unit Delay1/1, MinMax/1
  IPTc_v_PosCtrVoltRef1Max_back1/1 -> Subtract2/1
  Subtract2/1 -> Switch/3
  Unit Delay1/1 -> MinMax/2
  Switch/1 -> Relational Operator1/1
  Subtract1/1 -> Switch/1

== system BPN_lib/BPN/ActCurDiag/ChaCurDiag/ConDchMeanCurCal ==
  IPTd_i_CurSnr : Inport
  Constant : Constant  Value=100  OutDataTypeMode=uint16  OutDataTypeStr=uint16
  Constant1 : Constant  Value=BMS_Const_TickTm_s  OutDataTypeMode=single  OutDataTypeStr=single
  MeanCurCal : Subsystem
  Relational Operator4 : RelationalOperator  Operator===  LogicOutDataTypeMode=boolean  OutDataTypeStr=boolean
  Unit Delay : UnitDelay  SampleTime=-1
  counter : Subsystem  TreatAsAtomicUnit=on  RTWFcnName=counter  mask(counter){initial_value=1, counter_limit=100}
      mask prompts: initial_value "Initial_Counter_Value"
      mask help: The block is a counter.It counts from initial counter value until counter limit,then it will count from initial counter value.
      settings: AttributesFormatString=[INITIAL_VALUE=%<initial_value>]\n[COUNTER_LIMIT=%<counter_limit>]  RTWFcnNameOpts=User specified
      mask Display:
      | disp('COUNTER')
      | port_label('output',1,'out')
  gateway : Subsystem  TreatAsAtomicUnit=on
  iv=0.0 : Subsystem
  BPN_i_ConCurMean : Outport
  wires:
  Constant1/1 -> iv=0.0/3(dT)
  MeanCurCal/1(BPN_i_ConChaCur_Mean) -> BPN_i_ConCurMean/1
  IPTd_i_CurSnr/1 -> iv=0.0/2(u)
  gateway/1(Out1) -> MeanCurCal/1(BPN_i_ConChaCur1Sec_Mean)
  iv=0.0/1(yp) -> gateway/1(In1)
  Relational Operator4/1 -> gateway/Trigger, Unit Delay/1
  Constant/1 -> Relational Operator4/2
  counter/1(Out) -> Relational Operator4/1
  Unit Delay/1 -> MeanCurCal/Trigger, iv=0.0/1(R)

== system BPN_lib/BPN/ActCurDiag/DchCurDiag/ConDchMeanCurCal ==
  IPTd_i_CurSnr : Inport
  Constant : Constant  Value=100  OutDataTypeMode=uint16  OutDataTypeStr=uint16
  Constant1 : Constant  Value=BMS_Const_TickTm_s  OutDataTypeMode=single  OutDataTypeStr=single
  MeanCurCal : Subsystem
  Relational Operator4 : RelationalOperator  Operator===  LogicOutDataTypeMode=boolean  OutDataTypeStr=boolean
  Unit Delay : UnitDelay  SampleTime=-1
  counter : Subsystem  TreatAsAtomicUnit=on  RTWFcnName=counter  mask(counter){initial_value=1, counter_limit=150}
      mask prompts: initial_value "Initial_Counter_Value"
      mask help: The block is a counter.It counts from initial counter value until counter limit,then it will count from initial counter value.
      settings: AttributesFormatString=[INITIAL_VALUE=%<initial_value>]\n[COUNTER_LIMIT=%<counter_limit>]  RTWFcnNameOpts=User specified
      mask Display:
      | disp('COUNTER')
      | port_label('output',1,'out')
  gateway : Subsystem  TreatAsAtomicUnit=on
  iv=0.0 : Subsystem
  BPN_i_ConCurMean : Outport
  wires:
  Constant1/1 -> iv=0.0/3(dT)
  MeanCurCal/1(BPN_i_ConChaCur_Mean) -> BPN_i_ConCurMean/1
  IPTd_i_CurSnr/1 -> iv=0.0/2(u)
  gateway/1(Out1) -> MeanCurCal/1(BPN_i_ConChaCur1Sec_Mean)
  iv=0.0/1(yp) -> gateway/1(In1)
  Relational Operator4/1 -> gateway/Trigger, Unit Delay/1
  Constant/1 -> Relational Operator4/2
  counter/1(Out) -> Relational Operator4/1
  Unit Delay/1 -> MeanCurCal/Trigger, iv=0.0/1(R)

== system BPN_lib/BPN/PackVoltDropDiag/PackVoltDropDiag/MaxVoltMemoryMemory ==
  IPTd_v_PosCtrVoltRef1Max_front : Inport
  Enable : EnablePort
  IPTc_v_PosCtrVoltRef1Max_back : DataStoreWrite  DataStoreName=IPTc_v_PosCtrVoltRef1Max_front  SampleTime=-1
  wires:
  IPTd_v_PosCtrVoltRef1Max_front/1 -> IPTc_v_PosCtrVoltRef1Max_back/1

== system BPN_lib/BPN/ActCurDiag/ChaCurDiag/ConDchMeanCurCal/MeanCurCal ==
  BPN_i_ConChaCur1Sec_Mean : Inport
  Trigger : TriggerPort
  Constant : Constant  Value=100  OutDataTypeMode=single  OutDataTypeStr=single
  Divide : Product  Inputs=*/
  Sum of Elements : Sum  Inputs=+
  delay N=150s : Subsystem
  BPN_i_ConChaCur_Mean : Outport
  wires:
  Constant/1 -> Divide/2
  Divide/1 -> BPN_i_ConChaCur_Mean/1
  Sum of Elements/1 -> Divide/1
  delay N=150s/1(Out1) -> Sum of Elements/1
  BPN_i_ConChaCur1Sec_Mean/1 -> delay N=150s/1(In1)

== system BPN_lib/BPN/ActCurDiag/ChaCurDiag/ConDchMeanCurCal/counter ==
  counter : Stateflow chart  TreatAsAtomicUnit=on
  Out : Outport  OutDataType=fixdt(1, 16)  OutScaling=2^0
  wires:
  counter/1(out) -> Out/1

== system BPN_lib/BPN/ActCurDiag/ChaCurDiag/ConDchMeanCurCal/gateway ==
  In1 : Inport
  Trigger : TriggerPort
  Out1 : Outport
  wires:
  In1/1 -> Out1/1

== system BPN_lib/BPN/ActCurDiag/ChaCurDiag/ConDchMeanCurCal/iv=0.0 ==
  R : Inport
  u : Inport  Port=2
  dT : Inport  Port=3
  Add : Sum
  Fcn : Fcn  Expr=u^2
  Product : Product  RndMeth=Zero
  delay : Subsystem
  iv : Constant  Value=0
  yp : Outport
  wires:
  u/1 -> Fcn/1
  dT/1 -> Product/2
  Product/1 -> Add/1
  Fcn/1 -> Product/1
  delay/1(yp) -> yp/1
  delay/2(y) -> Add/2
  R/1 -> delay/2(R)
  iv/1 -> delay/3(iv)
  Add/1 -> delay/1(u)

== system BPN_lib/BPN/ActCurDiag/DchCurDiag/ConDchMeanCurCal/MeanCurCal ==
  BPN_i_ConChaCur1Sec_Mean : Inport
  Trigger : TriggerPort
  Constant : Constant  Value=150  OutDataTypeMode=single  OutDataTypeStr=single
  Divide : Product  Inputs=*/
  Sum of Elements : Sum  Inputs=+
  delay N=150s : Subsystem
  BPN_i_ConChaCur_Mean : Outport
  wires:
  Divide/1 -> BPN_i_ConChaCur_Mean/1
  Constant/1 -> Divide/2
  Sum of Elements/1 -> Divide/1
  delay N=150s/1(Out1) -> Sum of Elements/1
  BPN_i_ConChaCur1Sec_Mean/1 -> delay N=150s/1(In1)

== system BPN_lib/BPN/ActCurDiag/DchCurDiag/ConDchMeanCurCal/counter ==
  counter : Stateflow chart  TreatAsAtomicUnit=on
  Out : Outport  OutDataType=fixdt(1, 16)  OutScaling=2^0
  wires:
  counter/1(out) -> Out/1

== system BPN_lib/BPN/ActCurDiag/DchCurDiag/ConDchMeanCurCal/gateway ==
  In1 : Inport
  Trigger : TriggerPort
  Out1 : Outport
  wires:
  In1/1 -> Out1/1

== system BPN_lib/BPN/ActCurDiag/DchCurDiag/ConDchMeanCurCal/iv=0.0 ==
  R : Inport
  u : Inport  Port=2
  dT : Inport  Port=3
  Add : Sum
  Fcn : Fcn  Expr=u^2
  Product : Product  RndMeth=Zero
  delay : Subsystem
  iv : Constant  Value=0  OutDataTypeMode=single  OutDataTypeStr=single
  yp : Outport
  wires:
  u/1 -> Fcn/1
  dT/1 -> Product/2
  Product/1 -> Add/1
  Fcn/1 -> Product/1
  delay/1(yp) -> yp/1
  delay/2(y) -> Add/2
  R/1 -> delay/2(R)
  iv/1 -> delay/3(iv)
  Add/1 -> delay/1(u)

== system BPN_lib/BPN/ActCurDiag/ChaCurDiag/ConDchMeanCurCal/MeanCurCal/delay N=150s ==
  In1 : Inport
  Mux : Mux  Inputs=2
  Selector : Selector  InputPortWidth=151  IndexOptions=Index vector (dialog)  Indices=[2:151]  OutputSizes=1
  Unit Delay : UnitDelay  SampleTime=-1
  Out1 : Outport
  wires:
  In1/1 -> Mux/2
  Selector/1 -> Out1/1, Unit Delay/1
  Unit Delay/1 -> Mux/1
  Mux/1 -> Selector/1

== system BPN_lib/BPN/ActCurDiag/ChaCurDiag/ConDchMeanCurCal/iv=0.0/delay ==
  u : Inport
  R : Inport  Port=2  DataType=boolean  OutDataTypeStr=boolean
  iv : Inport  Port=3
  Logical Operator1 : Logic  Operator=NOT  AllPortsSameDT=off  OutDataTypeMode=boolean  OutDataTypeStr=boolean
  Switch2 : Switch  Criteria=u2 ~= 0
  Switch3 : Switch  Criteria=u2 ~= 0
  Unit Delay1 : UnitDelay  SampleTime=-1
  yp : Outport
  y : Outport  Port=2
  wires:
  u/1 -> Switch2/1
  Switch2/1 -> Unit Delay1/1, yp/1
  R/1 -> Switch3/2, Logical Operator1/1
  iv/1 -> Switch3/1
  Unit Delay1/1 -> Switch3/3, y/1
  Switch3/1 -> Switch2/3
  Logical Operator1/1 -> Switch2/2

== system BPN_lib/BPN/ActCurDiag/DchCurDiag/ConDchMeanCurCal/MeanCurCal/delay N=150s ==
  In1 : Inport
  Mux : Mux  Inputs=2
  Selector : Selector  InputPortWidth=151  IndexOptions=Index vector (dialog)  Indices=[2:151]  OutputSizes=1
  Unit Delay : UnitDelay  SampleTime=-1
  Out1 : Outport
  wires:
  In1/1 -> Mux/2
  Selector/1 -> Out1/1, Unit Delay/1
  Unit Delay/1 -> Mux/1
  Mux/1 -> Selector/1

== system BPN_lib/BPN/ActCurDiag/DchCurDiag/ConDchMeanCurCal/iv=0.0/delay ==
  u : Inport
  R : Inport  Port=2  DataType=boolean  OutDataTypeStr=boolean
  iv : Inport  Port=3
  Logical Operator1 : Logic  Operator=NOT  AllPortsSameDT=off  OutDataTypeMode=boolean  OutDataTypeStr=boolean
  Switch2 : Switch  Criteria=u2 ~= 0
  Switch3 : Switch  Criteria=u2 ~= 0
  Unit Delay1 : UnitDelay  SampleTime=-1
  yp : Outport
  y : Outport  Port=2
  wires:
  u/1 -> Switch2/1
  Switch2/1 -> Unit Delay1/1, yp/1
  R/1 -> Switch3/2, Logical Operator1/1
  iv/1 -> Switch3/1
  Unit Delay1/1 -> Switch3/3, y/1
  Switch3/1 -> Switch2/3
  Logical Operator1/1 -> Switch2/2

== stateflow chart BPN/CellVoltParamCalc/MaxVoltLocationCalc ==
  (default) -> (junction 3) : {j=0;}
  (junction 3) -> (junction 8) [order 2]
  (junction 6) -> (junction 5) [order 1] : [BPNd_v_CellVoltReshap[i][j] == BPNd_v_CellMaxVolt ]
      | {BPNd_enum_MaxVoltCellNum= ...
      | PACK_Const_CellNumOfMdl*j+i+1;
      | BPNd_enum_MaxVoltMdlNum=j+1;}
  (junction 3) -> (junction 6) [order 1] : [j<PACK_Const_MdlNumOfPack]
      | {i=0;}
  (junction 6) -> (junction 7) [order 2] : {i++;}
  (junction 7) -> (junction 6) [order 1] : [i<PACK_Const_CellNumOfMdl]
  (junction 4) -> (junction 3)
  (junction 7) -> (junction 4) [order 2] : {j++;}
  data: BPNd_v_CellMaxVolt input single; PACK_Const_CellNumOfMdl input uint8; i local uint8; j local uint8; PACK_Const_MdlNumOfPack input uint8; BPNd_enum_MaxVoltCellNum output uint8; BPNd_enum_MaxVoltMdlNum output uint8; BPNd_v_CellVoltReshap input single

== stateflow chart BPN/ActCurDiag/ChaCurDiag/ConDchMeanCurCal/counter/counter ==
  state COUNTER
    (default) -> (junction 28) : {counter=initial_value;}
    COUNTER -> (junction 28) [order 1]
    (junction 28) -> (junction 29) : {out=counter;counter+=1;}
  COUNTER -> (junction 30) [order 1] : [out>=counter_limit]
  (junction 30) -> (junction 31)
  (junction 31) -> COUNTER
  (default) -> COUNTER
  data: out output uint16; counter local uint16; initial_value parameter uint16; counter_limit parameter uint16

== stateflow chart BPN/ActCurDiag/DchCurDiag/ConDchMeanCurCal/counter/counter ==
  state COUNTER
    (default) -> (junction 46) : {counter=initial_value;}
    COUNTER -> (junction 46) [order 1]
    (junction 46) -> (junction 47) : {out=counter;counter+=1;}
  COUNTER -> (junction 48) [order 1] : [out>=counter_limit]
  (junction 48) -> (junction 49)
  (junction 49) -> COUNTER
  (default) -> COUNTER
  data: out output uint16; counter local uint16; initial_value parameter uint16; counter_limit parameter uint16

== stateflow chart BPN/CellVoltParamCalc/MinVoltLocationCalc ==
  (default) -> (junction 63) : {j=0;}
  (junction 63) -> (junction 68) [order 2]
  (junction 66) -> (junction 65) [order 1] : [BPNd_v_CellVoltReshap[i][j] == BPNd_v_CellMinVolt]
      | {BPNd_enum_MinVoltCellNum= ...
      | PACK_Const_CellNumOfMdl*j+i+1;
      | BPNd_enum_MinVoltMdlNum=j+1;}
  (junction 63) -> (junction 66) [order 1] : [j<PACK_Const_MdlNumOfPack]
      | {i=0;}
  (junction 66) -> (junction 67) [order 2] : {i++;}
  (junction 67) -> (junction 66) [order 1] : [i<PACK_Const_CellNumOfMdl]
  (junction 64) -> (junction 63)
  (junction 67) -> (junction 64) [order 2] : {j++;}
  data: BPNd_enum_MinVoltCellNum output uint8; PACK_Const_CellNumOfMdl input uint8; i local uint8; j local uint8; BPNd_enum_MinVoltMdlNum output uint8; PACK_Const_MdlNumOfPack input uint8; BPNd_v_CellVoltReshap input single size=[5 32]; BPNd_v_CellMinVolt input single

== matlab function BPN/CellVoltDiag/cell_volt_diagnostic ==
  data: IPTd_t_PackTemp input double; BPNd_iflt_CellUnderVolt_fatal output double; BPNd_iflt_CellOverVolt_fatal output double; BPNc_v_CellVoltUnder_fault input double; Umeasmin input double; Umeasmax input double; BPNc_v_CellVoltOver_fault input double; TiDelta input double; Xhighin input single; Xlowin input single; Xhigh output single; Xlow output single
function [BPNd_iflt_CellUnderVolt_fatal,BPNd_iflt_CellOverVolt_fatal,Xhigh,Xlow] = fcn(IPTd_t_PackTemp,BPNc_v_CellVoltUnder_fault,Umeasmin,Umeasmax,BPNc_v_CellVoltOver_fault,TiDelta,Xhighin,Xlowin)
%#eml
% inputs
Ti=IPTd_t_PackTemp;
dt=TiDelta;
Xhigh=single(0);
Xlow=single(0);
% different voltage limit at different temperature
Umax=4.15;
if Ti>=-20;
    Umin=2.7;
else
    Umin=2.1;
end

% different Xerr limit at different temperature
T=single([-25 -10]);
y=single([0.05 0.02]);
y1=single([0.45 0.8]);
if  Ti<= -10;
    if Ti>-25;
        Xerrhigh= interp1(T,y,Ti);
        Xerrlow= interp1(T,y1,Ti);
    else
    Xerrhigh=single(0.05);
    Xerrlow=single(0.45);
    end
else
    Xerrhigh=single(0.02);
    Xerrlow=single(0.8);
end   
%Umax Limit calculate input result
if Umeasmax>BPNc_v_CellVoltOver_fault
Xhigh=abs(Umeasmax-Umax)*(Umeasmax-Umax)*dt+Xhighin;
    if Xhigh> Xerrhigh
         BPNd_iflt_CellOverVolt_fatal=1;
         if Xhigh> Xerrhigh+1;
             Xhigh=single(1);
         else
            Xhigh=abs(Umeasmax-Umax)*(Umeasmax-Umax)*dt+Xhighin; 
         end
    else
         BPNd_iflt_CellOverVolt_fatal=0;
    end
else
      BPNd_iflt_CellOverVolt_fatal=0;
end  

%Umin Limit calculate and input result
if Umeasmin<BPNc_v_CellVoltUnder_fault;
Xlow=abs(Umin-Umeasmin)*(Umin-Umeasmin)*dt+Xlowin;
    if Xlow>Xerrlow;
          BPNd_iflt_CellUnderVolt_fatal=1;
          if Xlow>Xerrlow+1;
              Xlow=single(1);
          else 
            Xlow=abs(Umin-Umeasmin)*(Umin-Umeasmin)*dt+Xlowin;  
          end
    else
         BPNd_iflt_CellUnderVolt_fatal=0;
    end
else
    BPNd_iflt_CellUnderVolt_fatal=0;
end
